simulink model "test_mashinka_mapp_4"  (R2020b)
settings: Solver=ode45  StartTime=0.0  StopTime=20000  RelTol=1e-3  EnableMultiTasking=on
undefined symbols (not defined in the file): CMD_ci_Re_9, CMD_fb, CMD_Firprg_0, CMD_Firprg_1, CMD_gain, CMD_ind_mult, CMD_ind_mult_1, CMD_ind_mult_2, CMD_ind_mult_3, CMD_ind_mult_4, CMD_ind_vol, CMD_ind_vol_1, CMD_ind_vol_2, CMD_ind_vol_3, CMD_ind_vol_4, CMD_nl, CMD_param_0, CMD_pedal, CMD_reset, CMD_shape_0, CMD_step_down, CMD_step_up, ind_mult_0, ind_mult_1, ind_mult_2, ind_mult_3, ind_mult_4, ind_mult_multiplier, num_harm_0, num_pts0, num_str0, num_str1, Res, rom_length
libraries: xbsIndex_r4 x2299
(part 4 of 11)

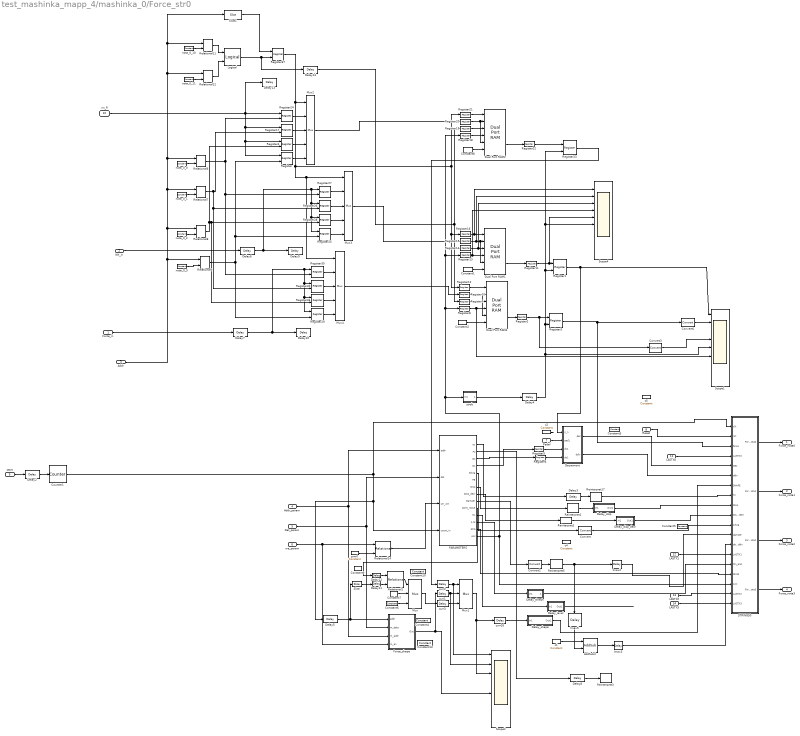
== system test_mashinka_mapp_4/mashinka_0/Force_str0 ==
  Force_in : Inport
  NN_in : Inport  Port=2
  Addr : Inport  Port=3
  Addr_param : Inport  Port=4
  Dat_param : Inport  Port=5
  we_param : Inport  Port=6
  Pedal : Inport  Port=7
  Reset : Inport  Port=8
  start : Inport  Port=9
  nn_fl : Inport  Port=10
  LASTX0 : Inport  Port=11
  LASTX1 : Inport  Port=12
  LASTX2 : Inport  Port=13
  LASTX3 : Inport  Port=14
  AddSub4 : xbsIndex_r4/AddSub  mode=Subtraction  use_carryin=off  use_carryout=off  en=off  latency=4  precision=User Defined  arith_type=Unsigned  n_bits=24  bin_pt=24  quantization=Truncate  overflow=Wrap  use_behavioral_HDL=on  hw_selection=Fabric  pipelined=off  use_rpm=on  dbl_ovrd=off  block_type=addsub
      settings: xl_area=[13 0 0 25 0 0 0]  block_version=VER_STRING_GOES_HERE
  Constant1 : xbsIndex_r4/Constant  const=0  gui_display_data_type=Boolean  arith_type=Boolean  n_bits=48  bin_pt=0  preci_type=Single  exp_width=8  frac_width=24  explicit_period=off  period=1  equ=P=C  opselect=C  inp2=PCIN>>17  opr=+  inp1=P  carry=CIN  dbl_ovrd=off  block_type=constant
      settings: block_version=VER_STRING_GOES_HERE
  Constant10 : xbsIndex_r4/Constant  const=1  gui_display_data_type=Fixed-point  arith_type=Unsigned  n_bits=1  bin_pt=0  preci_type=Single  exp_width=8  frac_width=24  explicit_period=on  period=1  equ=P=C  opselect=C  inp2=PCIN>>17  opr=+  inp1=P  carry=CIN  dbl_ovrd=off  block_type=constant
      settings: block_version=VER_STRING_GOES_HERE
  Constant13 : xbsIndex_r4/Constant  const=0  gui_display_data_type=Fixed-point  arith_type=Unsigned  n_bits=24  bin_pt=0  preci_type=Single  exp_width=8  frac_width=24  explicit_period=on  period=1  equ=P=C  opselect=C  inp2=PCIN>>17  opr=+  inp1=P  carry=CIN  dbl_ovrd=off  block_type=constant
      settings: block_version=VER_STRING_GOES_HERE
  Constant2 : xbsIndex_r4/Constant  const=0  gui_display_data_type=Boolean  arith_type=Boolean  n_bits=48  bin_pt=0  preci_type=Single  exp_width=8  frac_width=24  explicit_period=off  period=1  equ=P=C  opselect=C  inp2=PCIN>>17  opr=+  inp1=P  carry=CIN  dbl_ovrd=off  block_type=constant
      settings: block_version=VER_STRING_GOES_HERE
  Constant3 : xbsIndex_r4/Constant  const=0  gui_display_data_type=Boolean  arith_type=Boolean  n_bits=18  bin_pt=0  preci_type=Single  exp_width=8  frac_width=24  explicit_period=on  period=1  equ=P=C  opselect=C  inp2=PCIN>>17  opr=+  inp1=P  carry=CIN  dbl_ovrd=off  block_type=constant
      settings: block_version=VER_STRING_GOES_HERE
  Constant4 : xbsIndex_r4/Constant  const=100000  gui_display_data_type=Fixed-point  arith_type=Unsigned  n_bits=24  bin_pt=0  preci_type=Single  exp_width=8  frac_width=24  explicit_period=on  period=1  equ=P=C  opselect=C  inp2=PCIN>>17  opr=+  inp1=P  carry=CIN  dbl_ovrd=off  block_type=constant
      settings: block_version=VER_STRING_GOES_HERE
  Constant5 : xbsIndex_r4/Constant  const=1000  gui_display_data_type=Fixed-point  arith_type=Unsigned  n_bits=18  bin_pt=0  preci_type=Single  exp_width=8  frac_width=24  explicit_period=on  period=1  equ=P=C  opselect=C  inp2=PCIN>>17  opr=+  inp1=P  carry=CIN  dbl_ovrd=off  block_type=constant
      settings: block_version=VER_STRING_GOES_HERE
  Constant6 : xbsIndex_r4/Constant  const=1000  gui_display_data_type=Fixed-point  arith_type=Unsigned  n_bits=24  bin_pt=0  preci_type=Single  exp_width=8  frac_width=24  explicit_period=on  period=1  equ=P=C  opselect=C  inp2=PCIN>>17  opr=+  inp1=P  carry=CIN  dbl_ovrd=off  block_type=constant
      settings: block_version=VER_STRING_GOES_HERE
  Constant7 : xbsIndex_r4/Constant  const=0  gui_display_data_type=Fixed-point  arith_type=Unsigned  n_bits=24  bin_pt=0  preci_type=Single  exp_width=8  frac_width=24  explicit_period=on  period=1  equ=P=C  opselect=C  inp2=PCIN>>17  opr=+  inp1=P  carry=CIN  dbl_ovrd=off  block_type=constant
      settings: block_version=VER_STRING_GOES_HERE
  Constant8 : xbsIndex_r4/Constant  const=0  gui_display_data_type=Boolean  arith_type=Boolean  n_bits=48  bin_pt=0  preci_type=Single  exp_width=8  frac_width=24  explicit_period=off  period=1  equ=P=C  opselect=C  inp2=PCIN>>17  opr=+  inp1=P  carry=CIN  dbl_ovrd=off  block_type=constant
      settings: block_version=VER_STRING_GOES_HERE
  Constant9 : xbsIndex_r4/Constant  const=0  gui_display_data_type=Fixed-point  arith_type=Unsigned  n_bits=24  bin_pt=0  preci_type=Single  exp_width=8  frac_width=24  explicit_period=on  period=1  equ=P=C  opselect=C  inp2=PCIN>>17  opr=+  inp1=P  carry=CIN  dbl_ovrd=off  block_type=constant
      settings: block_version=VER_STRING_GOES_HERE
  Convert : xbsIndex_r4/Convert  gui_display_data_type=Fixed-point  arith_type=Unsigned  n_bits=9  bin_pt=0  float_type=Single  exp_bits=8  fraction_bits=24  quantization=Truncate  overflow=Wrap  en=off  latency=0  pipeline=off  dbl_ovrd=off  block_type=convert
  Convert2 : xbsIndex_r4/Convert  gui_display_data_type=Fixed-point  arith_type=Unsigned  n_bits=24  bin_pt=0  float_type=Single  exp_bits=8  fraction_bits=24  quantization=Truncate  overflow=Wrap  en=off  latency=0  pipeline=off  dbl_ovrd=off  block_type=convert
      settings: block_version=VER_STRING_GOES_HERE
  Convert3 : xbsIndex_r4/Convert  gui_display_data_type=Floating-point  arith_type=Floating-point  n_bits=16  bin_pt=14  float_type=Single  exp_bits=8  fraction_bits=24  quantization=Truncate  overflow=Wrap  en=off  latency=0  pipeline=off  dbl_ovrd=off  block_type=convert
  Convert6 : xbsIndex_r4/Convert  gui_display_data_type=Floating-point  arith_type=Floating-point  n_bits=16  bin_pt=14  float_type=Single  exp_bits=8  fraction_bits=24  quantization=Truncate  overflow=Wrap  en=off  latency=0  pipeline=off  dbl_ovrd=off  block_type=convert
  Counter1 : xbsIndex_r4/Counter  cnt_type=Count Limited  cnt_to=num_str0*(num_point_256) - 1  operation=Up  start_count=0  cnt_by_val=1  arith_type=Unsigned  n_bits=ceil(log2(num_str0*num_point_256))  bin_pt=0  load_pin=off  rst=off  en=on  explicit_period=on  period=1  use_behavioral_HDL=off  implementation=Fabric  use_rpm=off  dbl_ovrd=off  block_type=counter
      settings: block_version=8.2.02
  Decrement : Subsystem
  Delay10 : xbsIndex_r4/Delay  rst=off  infoeditControl=Selection of Reset will increase slice count due to use of real FFs and instead of SRLs  en=off  latency=5  reg_retiming=on  dbl_ovrd=off  block_type=delay
      settings: xl_area=[2 4 0 4 0 0 0]  block_version=8.2-EVAL
  Delay{2,6,11..12,14} (5 alike) : xbsIndex_r4/Delay  rst=off  infoeditControl=Selection of Reset will increase slice count due to use of real FFs and instead of SRLs  en=off  latency=1  reg_retiming=on  dbl_ovrd=off  block_type=delay
      settings: xl_area=[2 4 0 4 0 0 0]  block_version=8.2-EVAL
  Delay13 : xbsIndex_r4/Delay  rst=off  infoeditControl=Selection of Reset will increase slice count due to use of real FFs and instead of SRLs  en=off  latency=6  reg_retiming=on  dbl_ovrd=off  block_type=delay
      settings: xl_area=[2 4 0 4 0 0 0]  block_version=8.2-EVAL
  Delay3 : xbsIndex_r4/Delay  rst=off  infoeditControl=Selection of Reset will increase slice count due to use of real FFs and instead of SRLs  en=off  latency=29  reg_retiming=on  dbl_ovrd=off  block_type=delay
      settings: xl_area=[2 4 0 4 0 0 0]  block_version=8.2-EVAL
  Delay4 : xbsIndex_r4/Delay  rst=off  infoeditControl=Selection of Reset will increase slice count due to use of real FFs and instead of SRLs  en=off  latency=3  reg_retiming=on  dbl_ovrd=off  block_type=delay
      settings: xl_area=[2 4 0 4 0 0 0]  block_version=8.2-EVAL
  Delay5 : xbsIndex_r4/Delay  rst=off  infoeditControl=Selection of Reset will increase slice count due to use of real FFs and instead of SRLs  en=off  latency=23  reg_retiming=on  dbl_ovrd=off  block_type=delay
      settings: xl_area=[2 4 0 4 0 0 0]  block_version=8.2-EVAL
  Delay7 : xbsIndex_r4/Delay  rst=off  infoeditControl=Selection of Reset will increase slice count due to use of real FFs and instead of SRLs  en=off  latency=2  reg_retiming=on  dbl_ovrd=off  block_type=delay
      settings: xl_area=[2 4 0 4 0 0 0]  block_version=8.2-EVAL
  Delay8 : xbsIndex_r4/Delay  rst=off  infoeditControl=Selection of Reset will increase slice count due to use of real FFs and instead of SRLs  en=off  latency=28  reg_retiming=on  dbl_ovrd=off  block_type=delay
      settings: xl_area=[2 4 0 4 0 0 0]  block_version=8.2-EVAL
  Delay9 : xbsIndex_r4/Delay  rst=off  infoeditControl=Selection of Reset will increase slice count due to use of real FFs and instead of SRLs  en=off  latency=5  reg_retiming=on  dbl_ovrd=off  block_type=delay
      settings: xl_area=[2 4 0 4 0 0 0]  block_version=8.2-EVAL
  Delay_disp : Subsystem
  Delay_disp_decr : Subsystem
  Delay_level : Subsystem
  Delay_shape : Subsystem
  Delay_thresh : Subsystem
  Dual Port RAM1 : xbsIndex_r4/Dual Port RAM  depth=2^ceil(log2(num_str1))  initVector=zeros  distributed_mem=Block RAM  init_a=0  init_b=0  rst_a=off  rst_b=off  en_a=off  en_b=off  latency=1  write_mode_A=Read Before Write  write_mode_B=Read Before Write  optimize=Area  dbl_ovrd=off  simulation_type=fast_sim  block_type=dpram
      settings: block_version=10.1.1
  Dual Port RAM2 : xbsIndex_r4/Dual Port RAM  depth=2^ceil(log2(num_str1))  initVector=zeros  distributed_mem=Block RAM  init_a=0  init_b=0  rst_a=off  rst_b=off  en_a=off  en_b=off  latency=1  write_mode_A=Read Before Write  write_mode_B=Read Before Write  optimize=Area  dbl_ovrd=off  simulation_type=fast_sim  block_type=dpram
      settings: block_version=10.1.1
  Dual Port RAM4 : xbsIndex_r4/Dual Port RAM  depth=2^ceil(log2(num_str1))  initVector=zeros  distributed_mem=Block RAM  init_a=0  init_b=0  rst_a=off  rst_b=off  en_a=off  en_b=off  latency=1  write_mode_A=Read Before Write  write_mode_B=Read Before Write  optimize=Area  dbl_ovrd=off  simulation_type=fast_sim  block_type=dpram
      settings: block_version=10.1.1
  Force_shape : Subsystem
  Imax2 : xbsIndex_r4/Delay  rst=off  infoeditControl=Selection of Reset will increase slice count due to use of real FFs and instead of SRLs  en=off  latency=1  reg_retiming=on  dbl_ovrd=off  block_type=delay
      settings: xl_area=[12 24 0 0 0 0 0]  block_version=VER_STRING_GOES_HERE
  Imax3 : xbsIndex_r4/Delay  rst=off  infoeditControl=Selection of Reset will increase slice count due to use of real FFs and instead of SRLs  en=off  latency=1  reg_retiming=on  dbl_ovrd=off  block_type=delay
      settings: xl_area=[12 24 0 0 0 0 0]  block_version=VER_STRING_GOES_HERE
  Imax5 : xbsIndex_r4/Delay  rst=off  infoeditControl=Selection of Reset will increase slice count due to use of real FFs and instead of SRLs  en=off  latency=6  reg_retiming=on  dbl_ovrd=off  block_type=delay
      settings: infoedit=Hardware notes: A delay line is a chain, each link of which is an SRL16 followed by a flip-flop. If register retiming is enabled, the delay line is a chain of flip-flops.  xl_area=[12 24 0 24 0 0 0]  block_version=VER_STRING_GOES_HERE
  Logical : xbsIndex_r4/Logical  logical_function=AND  inputs=2  en=off  latency=0  precision=Full  arith_type=Unsigned  n_bits=16  bin_pt=0  align_bp=on  dbl_ovrd=off  block_type=logical
  Mux : xbsIndex_r4/Mux  inputs=2  en=off  latency=1  precision=Full  arith_type=Unsigned  n_bits=16  bin_pt=14  quantization=Truncate  overflow=Wrap  dbl_ovrd=off  block_type=mux
  Mux1 : xbsIndex_r4/Mux  inputs=2  en=off  latency=0  precision=Full  arith_type=Unsigned  n_bits=16  bin_pt=14  quantization=Truncate  overflow=Wrap  dbl_ovrd=off  block_type=mux
  Mux2 : xbsIndex_r4/Mux  inputs=4  en=off  latency=0  precision=Full  arith_type=Unsigned  n_bits=16  bin_pt=14  quantization=Truncate  overflow=Wrap  dbl_ovrd=off  block_type=mux
  Mux3 : xbsIndex_r4/Mux  inputs=4  en=off  latency=0  precision=Full  arith_type=Unsigned  n_bits=16  bin_pt=14  quantization=Truncate  overflow=Wrap  dbl_ovrd=off  block_type=mux
  Mux4 : xbsIndex_r4/Mux  inputs=4  en=off  latency=0  precision=Full  arith_type=Unsigned  n_bits=16  bin_pt=14  quantization=Truncate  overflow=Wrap  dbl_ovrd=off  block_type=mux
  PARAMETERS : Subsystem
  Register{,1,3..4,17,23..30,35..37} (16 alike) : xbsIndex_r4/Register  init=0  rst=off  en=on  dbl_ovrd=off  block_type=register
      Register1 settings: xl_area=[18 36 0 0 0 0 0]  block_version=VER_STRING_GOES_HERE
      Register23 settings: xl_area=[18 36 0 0 0 0 0]  block_version=VER_STRING_GOES_HERE
      Register3 settings: xl_area=[18 36 0 0 0 0 0]  block_version=VER_STRING_GOES_HERE
  Register{2,5..6,8..16,18..22} (17 alike) : xbsIndex_r4/Register  init=0  rst=off  en=off  dbl_ovrd=off  block_type=register
  Reinterpret{1..3,17} (4 alike) : xbsIndex_r4/Reinterpret  force_arith_type=off  arith_type="Signed  (2's comp)"  force_bin_pt=on  bin_pt=24  block_type=cast
      settings: block_version=VER_STRING_GOES_HERE
  Reinterpret5 : xbsIndex_r4/Reinterpret  force_arith_type=on  arith_type=Unsigned  force_bin_pt=on  bin_pt=24  block_type=cast
      settings: block_version=VER_STRING_GOES_HERE
  Relational{1,6..9,14} (6 alike) : xbsIndex_r4/Relational  mode=a=b  op_type=Bool  en=off  latency=0  dbl_ovrd=off  block_type=relational
      Relational6 settings: block_version=9.2.01
      Relational7 settings: block_version=9.2.01
      Relational8 settings: block_version=9.2.01
      Relational9 settings: block_version=9.2.01
  Relational11 : xbsIndex_r4/Relational  mode=a<=b  op_type=Bool  en=off  latency=0  dbl_ovrd=off  block_type=relational
      settings: block_version=9.2.01
  Relational12 : xbsIndex_r4/Relational  mode=a>b  op_type=Bool  en=off  latency=0  dbl_ovrd=off  block_type=relational
      settings: block_version=9.2.01
  STRINGS0 : Subsystem
  Scope1 : Scope  NumInputPorts=9
  Scope2 : Scope  NumInputPorts=8
  Scope4 : Scope  NumInputPorts=10
  Slice : xbsIndex_r4/Slice  nbits=8  boolean_output=off  mode=Lower Bit Location + Width  bit1=0  base1=MSB of Input  bit0=0  base0=LSB of Input  dbl_ovrd=off  block_type=slice
  Slice1 : xbsIndex_r4/Slice  nbits=2  boolean_output=off  mode=Lower Bit Location + Width  bit1=0  base1=MSB of Input  bit0=0  base0=LSB of Input  dbl_ovrd=off  block_type=slice
  c1 : xbsIndex_r4/Constant  const=1  gui_display_data_type=Fixed-point  arith_type=Unsigned  n_bits=24  bin_pt=23  preci_type=Single  exp_width=8  frac_width=24  explicit_period=off  period=1  equ=P=C  opselect=C  inp2=PCIN>>17  opr=+  inp1=P  carry=CIN  dbl_ovrd=off  block_type=constant
      settings: block_version=VER_STRING_GOES_HERE
  c2 : xbsIndex_r4/Constant  const=0  gui_display_data_type=Fixed-point  arith_type=Unsigned  n_bits=7  bin_pt=0  preci_type=Single  exp_width=8  frac_width=24  explicit_period=off  period=1  equ=P=C  opselect=C  inp2=PCIN>>17  opr=+  inp1=P  carry=CIN  dbl_ovrd=off  block_type=constant
      settings: block_version=VER_STRING_GOES_HERE
  c4 : xbsIndex_r4/Constant  const=200  gui_display_data_type=Fixed-point  arith_type=Unsigned  n_bits=8  bin_pt=0  preci_type=Single  exp_width=8  frac_width=24  explicit_period=on  period=1  equ=P=C  opselect=C  inp2=PCIN>>17  opr=+  inp1=P  carry=CIN  dbl_ovrd=off  block_type=constant
      settings: block_version=VER_STRING_GOES_HERE
  c5 : xbsIndex_r4/Constant  const=0  gui_display_data_type=Fixed-point  arith_type=Unsigned  n_bits=7  bin_pt=0  preci_type=Single  exp_width=8  frac_width=24  explicit_period=off  period=1  equ=P=C  opselect=C  inp2=PCIN>>17  opr=+  inp1=P  carry=CIN  dbl_ovrd=off  block_type=constant
      settings: block_version=VER_STRING_GOES_HERE
  curr{1..3,16} (4 alike) : xbsIndex_r4/Delay  rst=off  infoeditControl=Selection of Reset will increase slice count due to use of real FFs and instead of SRLs  en=off  latency=1  reg_retiming=on  dbl_ovrd=off  block_type=delay
      settings: xl_area=[17 33 0 33 0 0 0]  block_version=VER_STRING_GOES_HERE
  nota_0_0 : xbsIndex_r4/Constant  const=nota_0_0  gui_display_data_type=Fixed-point  arith_type=Unsigned  n_bits=7  bin_pt=0  preci_type=Single  exp_width=8  frac_width=24  explicit_period=on  period=1  equ=P=C  opselect=C  inp2=PCIN>>17  opr=+  inp1=P  carry=CIN  dbl_ovrd=off  block_type=constant
      settings: block_version=VER_STRING_GOES_HERE
  nota_0_1 : xbsIndex_r4/Constant  const=nota_0_1  gui_display_data_type=Fixed-point  arith_type=Unsigned  n_bits=7  bin_pt=0  preci_type=Single  exp_width=8  frac_width=24  explicit_period=on  period=1  equ=P=C  opselect=C  inp2=PCIN>>17  opr=+  inp1=P  carry=CIN  dbl_ovrd=off  block_type=constant
      settings: block_version=VER_STRING_GOES_HERE
  nota_0_10 : xbsIndex_r4/Constant  const=95  gui_display_data_type=Fixed-point  arith_type=Unsigned  n_bits=7  bin_pt=0  preci_type=Single  exp_width=8  frac_width=24  explicit_period=on  period=1  equ=P=C  opselect=C  inp2=PCIN>>17  opr=+  inp1=P  carry=CIN  dbl_ovrd=off  block_type=constant
      settings: block_version=VER_STRING_GOES_HERE
  nota_0_11 : xbsIndex_r4/Constant  const=91  gui_display_data_type=Fixed-point  arith_type=Unsigned  n_bits=7  bin_pt=0  preci_type=Single  exp_width=8  frac_width=24  explicit_period=on  period=1  equ=P=C  opselect=C  inp2=PCIN>>17  opr=+  inp1=P  carry=CIN  dbl_ovrd=off  block_type=constant
      settings: block_version=VER_STRING_GOES_HERE
  nota_0_2 : xbsIndex_r4/Constant  const=nota_0_2  gui_display_data_type=Fixed-point  arith_type=Unsigned  n_bits=7  bin_pt=0  preci_type=Single  exp_width=8  frac_width=24  explicit_period=on  period=1  equ=P=C  opselect=C  inp2=PCIN>>17  opr=+  inp1=P  carry=CIN  dbl_ovrd=off  block_type=constant
      settings: block_version=VER_STRING_GOES_HERE
  nota_0_3 : xbsIndex_r4/Constant  const=nota_0_3  gui_display_data_type=Fixed-point  arith_type=Unsigned  n_bits=7  bin_pt=0  preci_type=Single  exp_width=8  frac_width=24  explicit_period=on  period=1  equ=P=C  opselect=C  inp2=PCIN>>17  opr=+  inp1=P  carry=CIN  dbl_ovrd=off  block_type=constant
      settings: block_version=VER_STRING_GOES_HERE
  prm0 : xbsIndex_r4/Constant  const=prm0  gui_display_data_type=Fixed-point  arith_type=Unsigned  n_bits=8  bin_pt=0  preci_type=Single  exp_width=8  frac_width=24  explicit_period=on  period=1  equ=P=C  opselect=C  inp2=PCIN>>17  opr=+  inp1=P  carry=CIN  dbl_ovrd=off  block_type=constant
      settings: block_version=VER_STRING_GOES_HERE
  strob : Subsystem
  Force_nota0 : Outport  VectorParamsAs1DForOutWhenUnconnected=off
  Force_nota1 : Outport  Port=2  VectorParamsAs1DForOutWhenUnconnected=off
  Force_nota2 : Outport  Port=3  VectorParamsAs1DForOutWhenUnconnected=off
  Force_nota3 : Outport  Port=4  VectorParamsAs1DForOutWhenUnconnected=off
  wires:
  Mux/1 -> curr3/1
  strob/1(Out1) -> Delay4/1
  Register23/1 -> curr2/1
  Register22/1 -> Register23/1
  Dual Port RAM2/2 -> Register22/1
  Mux2/1 -> Register20/1
  Register21/1 -> Dual Port RAM2/1
  Register20/1 -> Dual Port RAM2/5, Dual Port RAM2/2
  Register19/1 -> Dual Port RAM2/3
  Constant8/1 -> Dual Port RAM2/6
  nn_fl/1 -> Register/1, Register4/1, Register17/1, Delay13/1, Register24/1
  curr3/1 -> Mux1/3
  curr1/1 -> Mux1/2, Scope2/2
  curr2/1 -> Mux1/1, Scope2/1
  curr16/1 -> Delay_shape/1(In1)
  Slice/1 -> Delay11/1
  Delay12/1 -> Relational1/1
  Constant7/1 -> Mux/2
  Constant6/1 -> Mux/3
  Relational1/1 -> Mux/1
  PARAMETERS/10(point_noise) -> Delay12/1
  Delay11/1 -> Relational1/2
  PARAMETERS/11(NL) -> Delay_level/1(In1)
  LASTX1/1 -> STRINGS0/14(LASTX1)
  Mux4/1 -> Register10/1
  NN_in/1 -> Delay6/1
  Convert/1 -> STRINGS0/11(sdvig)
  PARAMETERS/2(Fo) -> Delay8/1
  Delay8/1 -> Reinterpret3/1
  PARAMETERS/14(Acc) -> STRINGS0/17(Acc), Register13/1, Register18/1, Register8/1, strob/1(In1)
  Constant1/1 -> Dual Port RAM1/6
  Constant2/1 -> Dual Port RAM4/6
  Dual Port RAM4/2 -> Register2/1
  Delay14/1 -> Register9/1, Register14/1, Register19/1
  c2/1 -> ?
  PARAMETERS/4(Dc) -> Register5/1
  PARAMETERS/3(Do) -> Register6/1
  Dual Port RAM1/2 -> Register11/1
  Decrement/1(dec) -> STRINGS0/5(Dec)
  PARAMETERS/7(Disp) -> Reinterpret1/1
  PARAMETERS/8(Disp_decr) -> Reinterpret2/1
  Mux1/1 -> Scope2/3, curr16/1
  Reinterpret17/1 -> STRINGS0/8(Tn)
  Reinterpret1/1 -> Delay_disp/1(In1)
  Reinterpret2/1 -> Delay_disp_decr/1(In1)
  PARAMETERS/1(Tn) -> Delay3/1
  Delay3/1 -> Reinterpret17/1
  Decrement/2(ddiv) -> STRINGS0/6(ddiv)
  PARAMETERS/5(Sdvig) -> Convert/1
  Addr_param/1 -> Force_shape/3(m_addr), PARAMETERS/1(addr)
  Dat_param/1 -> Force_shape/2(m_data), PARAMETERS/2(dat)
  we_param/1 -> Relational14/1, Force_shape/4(m_en)
  Pedal/1 -> Decrement/2(ped1)
  Reset/1 -> STRINGS0/2(rst)
  LASTX0/1 -> STRINGS0/4(LASTX0)
  Force_in/1 -> Delay7/1
  Delay5/1 -> Force_shape/1(addr), Slice/1
  Register11/1 -> Scope4/5, Register1/1
  Register2/1 -> Convert3/1, Register3/1
  Register5/1 -> Decrement/3(dc1)
  Register6/1 -> Decrement/4(do1)
  Register1/1 -> Decrement/1(n_n), Scope1/1
  Register8/1 -> Scope1/6, Dual Port RAM4/4
  Register10/1 -> Dual Port RAM4/2, Dual Port RAM4/5
  Register12/1 -> Dual Port RAM4/1
  Register13/1 -> Dual Port RAM1/4, Scope4/4
  Register14/1 -> Scope4/3, Dual Port RAM1/3
  Register15/1 -> Scope4/2, Dual Port RAM1/2, Dual Port RAM1/5
  Register16/1 -> Scope4/1, Dual Port RAM1/1
  Convert2/1 -> Reinterpret5/1
  AddSub4/1 -> Imax3/1
  c1/1 -> AddSub4/1
  Reinterpret5/1 -> Imax5/1, Imax2/1
  Imax5/1 -> AddSub4/2
  Imax2/1 -> STRINGS0/12(damper)
  Imax3/1 -> STRINGS0/13(damper_ddiv)
  PARAMETERS/9(Damper) -> Convert2/1
  prm0/1 -> Relational14/2
  Relational14/1 -> PARAMETERS/3(str_we)
  Delay2/1 -> Counter1/1
  start/1 -> Delay2/1
  PARAMETERS/12(1-Nl) -> Delay_thresh/1(In1)
  Delay_thresh/1(ttn_end) -> STRINGS0/15(ttn_end)
  Delay_level/1(Out1) -> ?
  Delay_disp/1(Out1) -> STRINGS0/9(Disp)
  Delay_disp_decr/1(Out1) -> STRINGS0/10(Disp_decr)
  Delay_shape/1(Out1) -> STRINGS0/7(SHAPE)
  Mux3/1 -> Register15/1
  Register3/1 -> STRINGS0/3(force), Convert6/1
  Force_shape/1(Out) -> curr1/1, Scope2/5
  Register37/1 -> Mux4/1, Mux3/1, Register12/1, Register16/1, Register21/1, Mux2/1
  Register9/1 -> Dual Port RAM4/3
  PARAMETERS/13(Strb) -> STRINGS0/16(Strob)
  Register18/1 -> Dual Port RAM2/4
  Delay4/1 -> Scope1/5, Register1/2, Scope4/6, Register23/2, Register3/2
  Counter1/1 -> Delay5/1, PARAMETERS/4(count_in), STRINGS0/1(clk)
  STRINGS0/2(Force_nota1) -> Force_nota1/1
  STRINGS0/1(Force_nota0) -> Force_nota0/1
  STRINGS0/3(Force_nota2) -> Force_nota2/1
  STRINGS0/4(Force_nota3) -> Force_nota3/1
  LASTX2/1 -> STRINGS0/18(LASTX2)
  LASTX3/1 -> STRINGS0/19(LASTX3)
  Convert6/1 -> Scope1/2
  Convert3/1 -> Scope1/4
  nota_0_2/1 -> Relational8/2
  nota_0_3/1 -> Relational9/2
  nota_0_1/1 -> Relational7/2
  nota_0_0/1 -> Relational6/2
  Delay7/1 -> Register30/1, Register36/1, Register29/1, Register35/1, Delay10/1
  Relational6/1 -> Register35/2, Register27/2, Register24/2
  Relational7/1 -> Register30/2, Register26/2, Register17/2
  Relational8/1 -> Register36/2, Register28/2, Register4/2
  Relational9/1 -> Register29/2, Register25/2, Register/2
  Register24/1 -> Mux2/2
  Register17/1 -> Mux2/3
  Register4/1 -> Mux2/4
  Register/1 -> Mux2/5
  Register27/1 -> Mux3/2
  Register26/1 -> Mux3/3
  Register28/1 -> Mux3/4
  Register25/1 -> Mux3/5
  Register35/1 -> Mux4/2
  Register30/1 -> Mux4/3
  Register36/1 -> Mux4/4
  Register29/1 -> Mux4/5
  nota_0_10/1 -> Relational11/2
  nota_0_11/1 -> Relational12/2
  Addr/1 -> Slice1/1, Relational11/1, Relational12/1, Relational6/1, Relational7/1, Relational8/1, Relational9/1
  Relational11/1 -> Logical/1
  Relational12/1 -> Logical/2
  Logical/1 -> Delay14/1, Register37/2
  Slice1/1 -> Register37/1
  Delay6/1 -> Register26/1, Register28/1, Register25/1, Register27/1, Delay9/1

== system test_mashinka_mapp_4/Mid_Graph1/Exp/exp-mashinka ==
  Force_vol : Inport
  m_data : Inport  Port=2
  m_addr : Inport  Port=3
  m_en : Inport  Port=4
  Addr_ind_vol : Inport  Port=5
  Addr_sync : Inport  Port=6
  AddSub : xbsIndex_r4/AddSub  mode=Addition  use_carryin=off  use_carryout=off  en=off  latency=8  precision=Full  arith_type=Unsigned  n_bits=16  bin_pt=14  quantization=Truncate  overflow=Wrap  use_behavioral_HDL=off  hw_selection=Fabric  pipelined=off  dbl_ovrd=off  block_type=addsub
  AddSub1 : xbsIndex_r4/AddSub  mode=Addition  use_carryin=off  use_carryout=off  en=off  latency=8  precision=Full  arith_type=Unsigned  n_bits=16  bin_pt=14  quantization=Truncate  overflow=Wrap  use_behavioral_HDL=off  hw_selection=Fabric  pipelined=off  dbl_ovrd=off  block_type=addsub
  AddSub2 : xbsIndex_r4/AddSub  mode=Addition  use_carryin=off  use_carryout=off  en=off  latency=8  precision=Full  arith_type=Unsigned  n_bits=16  bin_pt=14  quantization=Truncate  overflow=Wrap  use_behavioral_HDL=off  hw_selection=Fabric  pipelined=off  dbl_ovrd=off  block_type=addsub
  Constant : xbsIndex_r4/Constant  const=0  gui_display_data_type=Fixed-point  arith_type=Unsigned  n_bits=30  bin_pt=0  preci_type=Single  exp_width=8  frac_width=24  explicit_period=on  period=1  equ=P=C  opselect=C  inp2=PCIN>>17  opr=+  inp1=P  carry=CIN  dbl_ovrd=off  block_type=constant
  Convert5 : xbsIndex_r4/Convert  gui_display_data_type=Floating-point  arith_type=Floating-point  n_bits=16  bin_pt=14  float_type=Single  exp_bits=8  fraction_bits=24  quantization=Truncate  overflow=Wrap  en=off  latency=0  pipeline=off  dbl_ovrd=off  block_type=convert
  Convert6 : xbsIndex_r4/Convert  gui_display_data_type=Floating-point  arith_type=Floating-point  n_bits=16  bin_pt=14  float_type=Single  exp_bits=8  fraction_bits=24  quantization=Truncate  overflow=Wrap  en=off  latency=0  pipeline=off  dbl_ovrd=off  block_type=convert
  Convert7 : xbsIndex_r4/Convert  gui_display_data_type=Floating-point  arith_type=Floating-point  n_bits=16  bin_pt=14  float_type=Single  exp_bits=8  fraction_bits=24  quantization=Truncate  overflow=Wrap  en=off  latency=0  pipeline=off  dbl_ovrd=off  block_type=convert
  Delay : xbsIndex_r4/Delay  rst=off  infoeditControl=Selection of Reset will increase slice count due to use of real FFs and instead of SRLs  en=off  latency=50  reg_retiming=off  dbl_ovrd=off  block_type=delay
  Delay1 : xbsIndex_r4/Delay  rst=off  infoeditControl=Selection of Reset will increase slice count due to use of real FFs and instead of SRLs  en=off  latency=1  reg_retiming=off  dbl_ovrd=off  block_type=delay
  Delay11 : xbsIndex_r4/Delay  rst=off  infoeditControl=Selection of Reset will increase slice count due to use of real FFs and instead of SRLs  en=off  latency=1  reg_retiming=off  dbl_ovrd=off  block_type=delay
  Delay2 : xbsIndex_r4/Delay  rst=off  infoeditControl=Selection of Reset will increase slice count due to use of real FFs and instead of SRLs  en=off  latency=1  reg_retiming=off  dbl_ovrd=off  block_type=delay
  Relational : xbsIndex_r4/Relational  mode=a!=b  op_type=Bool  en=off  latency=1  dbl_ovrd=off  block_type=relational
  Scope3 : Scope  NumInputPorts=10
  gauss0 : Subsystem
  gauss1 : Subsystem
  gauss2 : Subsystem
  gauss3 : Subsystem
  z12 : xbsIndex_r4/Delay  rst=off  infoeditControl=Selection of Reset will increase slice count due to use of real FFs and instead of SRLs  en=off  latency=1  reg_retiming=on  dbl_ovrd=off  block_type=delay
      settings: block_version=8.2-EVAL
  z9 : xbsIndex_r4/Delay  rst=off  infoeditControl=Selection of Reset will increase slice count due to use of real FFs and instead of SRLs  en=off  latency=1  reg_retiming=on  dbl_ovrd=off  block_type=delay
      settings: block_version=8.2-EVAL
  Out : Outport  VectorParamsAs1DForOutWhenUnconnected=off
  wires:
  AddSub2/1 -> Delay1/1
  Delay1/1 -> AddSub1/2
  gauss3/1(Out1) -> AddSub2/2
  gauss2/1(Out1) -> AddSub2/1
  gauss1/1(Out1) -> AddSub/2
  Convert7/1 -> Scope3/7
  Convert5/1 -> Scope3/5
  AddSub1/1 -> Delay2/1, Convert7/1
  AddSub/1 -> Delay11/1
  Delay11/1 -> Convert5/1, AddSub1/1
  gauss0/1(Out1) -> Convert6/1, AddSub/1
  z9/1 -> gauss0/7(Addr_ind_vol), gauss2/7(Addr_ind_vol), gauss3/7(Addr_ind_vol), gauss1/7(Addr_ind_vol)
  m_en/1 -> gauss0/6(m_en), gauss2/6(m_en), gauss3/6(m_en), gauss1/6(m_en)
  m_addr/1 -> gauss0/5(m_addr), gauss2/5(m_addr), gauss3/5(m_addr), gauss1/5(m_addr)
  m_data/1 -> gauss0/4(m_data), gauss2/4(m_data), gauss3/4(m_data), gauss1/4(m_data)
  Force_vol/1 -> gauss2/3(Force_vol), gauss3/3(Force_vol), gauss1/3(Force_vol), gauss0/3(Force_vol)
  Delay/1 -> gauss2/1(sync), gauss3/1(sync), gauss1/1(sync), gauss0/1(sync)
  z12/1 -> Relational/1, gauss0/2(addr), gauss2/2(addr), gauss3/2(addr), gauss1/2(addr)
  Delay2/1 -> Out/1
  Convert6/1 -> Scope3/1
  Relational/1 -> Delay/1
  Constant/1 -> Relational/2
  Addr_ind_vol/1 -> z9/1
  Addr_sync/1 -> z12/1

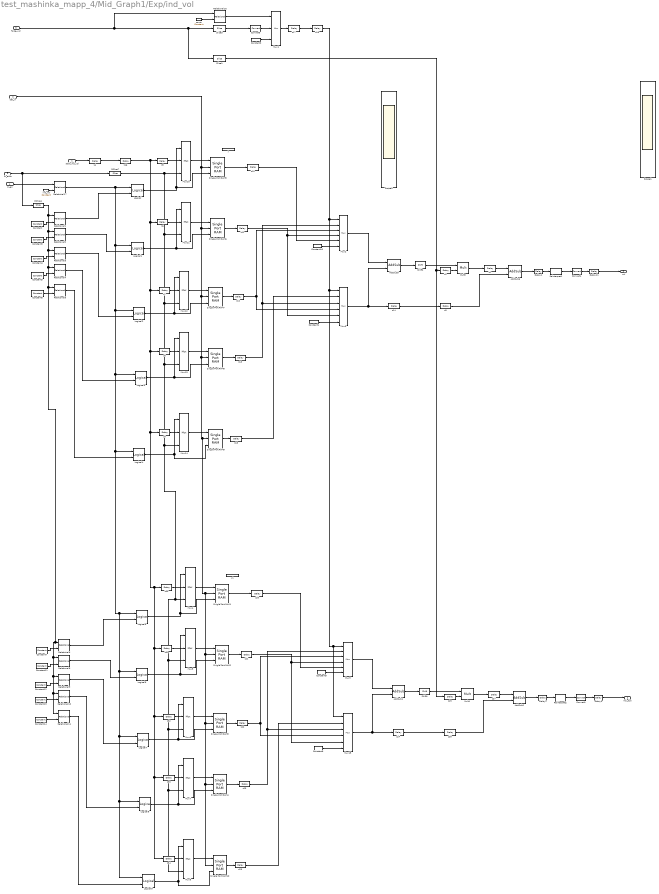
== system test_mashinka_mapp_4/Mid_Graph1/Exp/ind_vol ==
  addr_ind_vol : Inport
  dat_in : Inport  Port=2
  m_addr : Inport  Port=3
  m_en : Inport  Port=4
  force_vol : Inport  Port=5
  AddSub1 : xbsIndex_r4/AddSub  mode=Subtraction  use_carryin=off  use_carryout=off  en=off  latency=2  precision=Full  arith_type="Signed  (2's comp)"  n_bits=24  bin_pt=0  quantization=Truncate  overflow=Wrap  use_behavioral_HDL=off  hw_selection=Fabric  pipelined=off  dbl_ovrd=off  block_type=addsub
  AddSub2 : xbsIndex_r4/AddSub  mode=Addition  use_carryin=off  use_carryout=off  en=off  latency=2  precision=Full  arith_type=Unsigned  n_bits=24  bin_pt=0  quantization=Truncate  overflow=Wrap  use_behavioral_HDL=off  hw_selection=Fabric  pipelined=off  dbl_ovrd=off  block_type=addsub
  AddSub5 : xbsIndex_r4/AddSub  mode=Subtraction  use_carryin=off  use_carryout=off  en=off  latency=2  precision=Full  arith_type="Signed  (2's comp)"  n_bits=24  bin_pt=0  quantization=Truncate  overflow=Wrap  use_behavioral_HDL=off  hw_selection=Fabric  pipelined=off  dbl_ovrd=off  block_type=addsub
  AddSub6 : xbsIndex_r4/AddSub  mode=Addition  use_carryin=off  use_carryout=off  en=off  latency=2  precision=Full  arith_type=Unsigned  n_bits=24  bin_pt=0  quantization=Truncate  overflow=Wrap  use_behavioral_HDL=off  hw_selection=Fabric  pipelined=off  dbl_ovrd=off  block_type=addsub
  Constant : xbsIndex_r4/Constant  const=4  gui_display_data_type=Fixed-point  arith_type=Unsigned  n_bits=3  bin_pt=0  preci_type=Single  exp_width=8  frac_width=24  explicit_period=off  period=1  equ=P=C  opselect=C  inp2=PCIN>>17  opr=+  inp1=P  carry=CIN  dbl_ovrd=off  block_type=constant
  Constant{1,8..10} (4 alike) : xbsIndex_r4/Constant  const=0  gui_display_data_type=Fixed-point  arith_type=Unsigned  n_bits=24  bin_pt=0  preci_type=Single  exp_width=8  frac_width=24  explicit_period=on  period=1  equ=P=C  opselect=C  inp2=PCIN>>17  opr=+  inp1=P  carry=CIN  dbl_ovrd=off  block_type=constant
      settings: block_version=VER_STRING_GOES_HERE
  Constant11 : xbsIndex_r4/Constant  const=8  gui_display_data_type=Fixed-point  arith_type=Unsigned  n_bits=4  bin_pt=0  preci_type=Single  exp_width=8  frac_width=24  explicit_period=off  period=1  equ=P=C  opselect=C  inp2=PCIN>>17  opr=+  inp1=P  carry=CIN  dbl_ovrd=off  block_type=constant
  Constant12 : xbsIndex_r4/Constant  const=7  gui_display_data_type=Fixed-point  arith_type=Unsigned  n_bits=4  bin_pt=0  preci_type=Single  exp_width=8  frac_width=24  explicit_period=off  period=1  equ=P=C  opselect=C  inp2=PCIN>>17  opr=+  inp1=P  carry=CIN  dbl_ovrd=off  block_type=constant
  Constant13 : xbsIndex_r4/Constant  const=6  gui_display_data_type=Fixed-point  arith_type=Unsigned  n_bits=4  bin_pt=0  preci_type=Single  exp_width=8  frac_width=24  explicit_period=off  period=1  equ=P=C  opselect=C  inp2=PCIN>>17  opr=+  inp1=P  carry=CIN  dbl_ovrd=off  block_type=constant
  Constant14 : xbsIndex_r4/Constant  const=5  gui_display_data_type=Fixed-point  arith_type=Unsigned  n_bits=4  bin_pt=0  preci_type=Single  exp_width=8  frac_width=24  explicit_period=off  period=1  equ=P=C  opselect=C  inp2=PCIN>>17  opr=+  inp1=P  carry=CIN  dbl_ovrd=off  block_type=constant
  Constant2 : xbsIndex_r4/Constant  const=4  gui_display_data_type=Fixed-point  arith_type=Unsigned  n_bits=3  bin_pt=0  preci_type=Single  exp_width=8  frac_width=24  explicit_period=on  period=1  equ=P=C  opselect=C  inp2=PCIN>>17  opr=+  inp1=P  carry=CIN  dbl_ovrd=off  block_type=constant
      settings: block_version=VER_STRING_GOES_HERE
  Constant3 : xbsIndex_r4/Constant  const=3  gui_display_data_type=Fixed-point  arith_type=Unsigned  n_bits=3  bin_pt=0  preci_type=Single  exp_width=8  frac_width=24  explicit_period=off  period=1  equ=P=C  opselect=C  inp2=PCIN>>17  opr=+  inp1=P  carry=CIN  dbl_ovrd=off  block_type=constant
  Constant4 : xbsIndex_r4/Constant  const=2  gui_display_data_type=Fixed-point  arith_type=Unsigned  n_bits=3  bin_pt=0  preci_type=Single  exp_width=8  frac_width=24  explicit_period=off  period=1  equ=P=C  opselect=C  inp2=PCIN>>17  opr=+  inp1=P  carry=CIN  dbl_ovrd=off  block_type=constant
  Constant5 : xbsIndex_r4/Constant  const=1  gui_display_data_type=Fixed-point  arith_type=Unsigned  n_bits=3  bin_pt=0  preci_type=Single  exp_width=8  frac_width=24  explicit_period=off  period=1  equ=P=C  opselect=C  inp2=PCIN>>17  opr=+  inp1=P  carry=CIN  dbl_ovrd=off  block_type=constant
  Constant6 : xbsIndex_r4/Constant  const=0  gui_display_data_type=Fixed-point  arith_type=Unsigned  n_bits=3  bin_pt=0  preci_type=Single  exp_width=8  frac_width=24  explicit_period=off  period=1  equ=P=C  opselect=C  inp2=PCIN>>17  opr=+  inp1=P  carry=CIN  dbl_ovrd=off  block_type=constant
  Constant7 : xbsIndex_r4/Constant  const=9  gui_display_data_type=Fixed-point  arith_type=Unsigned  n_bits=4  bin_pt=0  preci_type=Single  exp_width=8  frac_width=24  explicit_period=off  period=1  equ=P=C  opselect=C  inp2=PCIN>>17  opr=+  inp1=P  carry=CIN  dbl_ovrd=off  block_type=constant
  Convert1 : xbsIndex_r4/Convert  gui_display_data_type=Floating-point  arith_type=Floating-point  n_bits=16  bin_pt=14  float_type=Single  exp_bits=8  fraction_bits=24  quantization=Truncate  overflow=Wrap  en=off  latency=3  pipeline=off  dbl_ovrd=off  block_type=convert
  Convert4 : xbsIndex_r4/Convert  gui_display_data_type=Floating-point  arith_type=Floating-point  n_bits=16  bin_pt=14  float_type=Single  exp_bits=8  fraction_bits=24  quantization=Truncate  overflow=Wrap  en=off  latency=3  pipeline=off  dbl_ovrd=off  block_type=convert
  Convert5 : xbsIndex_r4/Convert  gui_display_data_type=Fixed-point  arith_type=Unsigned  n_bits=3  bin_pt=0  float_type=Single  exp_bits=8  fraction_bits=24  quantization=Truncate  overflow=Wrap  en=off  latency=0  pipeline=off  dbl_ovrd=off  block_type=convert
  Delay{1..3,11} (4 alike) : xbsIndex_r4/Delay  rst=off  infoeditControl=Selection of Reset will increase slice count due to use of real FFs and instead of SRLs  en=off  latency=1  reg_retiming=off  dbl_ovrd=off  block_type=delay
  Logical{,1..9} (10 alike) : xbsIndex_r4/Logical  logical_function=AND  inputs=2  en=off  latency=1  precision=Full  arith_type=Unsigned  n_bits=16  bin_pt=0  align_bp=on  dbl_ovrd=off  block_type=logical
  Mult1 : xbsIndex_r4/Mult  precision=Full  arith_type="Signed  (2's comp)"  n_bits=16  bin_pt=14  quantization=Truncate  overflow=Wrap  en=off  latency=3  use_behavioral_HDL=off  opt=Speed  use_embedded=on  optimum_pipeline=off  pipeline=on  dbl_ovrd=off  use_rpm=on  placement_style=Triangular  block_type=mult
  Mult3 : xbsIndex_r4/Mult  precision=Full  arith_type="Signed  (2's comp)"  n_bits=16  bin_pt=14  quantization=Truncate  overflow=Wrap  en=off  latency=3  use_behavioral_HDL=off  opt=Speed  use_embedded=on  optimum_pipeline=off  pipeline=on  dbl_ovrd=off  use_rpm=on  placement_style=Triangular  block_type=mult
  Mux{1,4..8,10..14} (11 alike) : xbsIndex_r4/Mux  inputs=2  en=off  latency=0  precision=Full  arith_type=Unsigned  n_bits=16  bin_pt=14  quantization=Truncate  overflow=Wrap  dbl_ovrd=off  block_type=mux
  Mux{2..3,9,15} (4 alike) : xbsIndex_r4/Mux  inputs=5  en=off  latency=1  precision=Full  arith_type=Unsigned  n_bits=16  bin_pt=14  quantization=Truncate  overflow=Wrap  dbl_ovrd=off  block_type=mux
  RSlice1 : xbsIndex_r4/Slice  nbits=4  boolean_output=off  mode=Upper Bit Location + Width  bit1=0  base1=MSB of Input  bit0=0  base0=LSB of Input  dbl_ovrd=off  block_type=slice
      settings: block_version=VER_STRING_GOES_HERE
  RSlice7 : xbsIndex_r4/Slice  nbits=7  boolean_output=off  mode=Lower Bit Location + Width  bit1=0  base1=MSB of Input  bit0=0  base0=LSB of Input  dbl_ovrd=off  block_type=slice
      settings: block_version=VER_STRING_GOES_HERE
  Reinterpret1 : xbsIndex_r4/Reinterpret  force_arith_type=on  arith_type="Signed  (2's comp)"  force_bin_pt=on  bin_pt=24  block_type=reinterpret
  Reinterpret2 : xbsIndex_r4/Reinterpret  force_arith_type=on  arith_type="Signed  (2's comp)"  force_bin_pt=on  bin_pt=24  block_type=reinterpret
  Relational{1..6,8..11,16..17} (12 alike) : xbsIndex_r4/Relational  mode=a=b  op_type=Bool  en=off  latency=0  dbl_ovrd=off  block_type=relational
  Scope1 : Scope  NumInputPorts=8
  Scope3 : Scope  NumInputPorts=10
  Shift1 : xbsIndex_r4/Shift  shift_dir=Right  shift_bits=5  en=off  latency=0  precision=Full  arith_type="Signed  (2's comp)"  n_bits=16  bin_pt=14  quantization=Truncate  overflow=Wrap  dbl_ovrd=off  block_type=shift
  Shift2 : xbsIndex_r4/Shift  shift_dir=Right  shift_bits=5  en=off  latency=0  precision=Full  arith_type="Signed  (2's comp)"  n_bits=16  bin_pt=14  quantization=Truncate  overflow=Wrap  dbl_ovrd=off  block_type=shift
  Single Port RAM1 : xbsIndex_r4/Single Port RAM  depth=96  initVector=ind_vol_4  distributed_mem=Block RAM  write_mode=Read After Write  rst=off  init_reg=0  en=off  optimize_latency=off  latency=1  optimize=Area  dbl_ovrd=off  simulation_type=fast_sim  block_type=spram
  Single Port RAM10 : xbsIndex_r4/Single Port RAM  depth=96  initVector=ind_vol_0  distributed_mem=Block RAM  write_mode=Read After Write  rst=off  init_reg=0  en=off  optimize_latency=off  latency=1  optimize=Area  dbl_ovrd=off  simulation_type=fast_sim  block_type=spram
  Single Port RAM2 : xbsIndex_r4/Single Port RAM  depth=96  initVector=ind_vol_3  distributed_mem=Block RAM  write_mode=Read After Write  rst=off  init_reg=0  en=off  optimize_latency=off  latency=1  optimize=Area  dbl_ovrd=off  simulation_type=fast_sim  block_type=spram
  Single Port RAM3 : xbsIndex_r4/Single Port RAM  depth=96  initVector=ind_vol_2  distributed_mem=Block RAM  write_mode=Read After Write  rst=off  init_reg=0  en=off  optimize_latency=off  latency=1  optimize=Area  dbl_ovrd=off  simulation_type=fast_sim  block_type=spram
  Single Port RAM4 : xbsIndex_r4/Single Port RAM  depth=96  initVector=ind_vol_1  distributed_mem=Block RAM  write_mode=Read After Write  rst=off  init_reg=0  en=off  optimize_latency=off  latency=1  optimize=Area  dbl_ovrd=off  simulation_type=fast_sim  block_type=spram
  Single Port RAM5 : xbsIndex_r4/Single Port RAM  depth=96  initVector=ind_vol_4  distributed_mem=Block RAM  write_mode=Read After Write  rst=off  init_reg=0  en=off  optimize_latency=off  latency=1  optimize=Area  dbl_ovrd=off  simulation_type=fast_sim  block_type=spram
  Single Port RAM6 : xbsIndex_r4/Single Port RAM  depth=96  initVector=ind_vol_3  distributed_mem=Block RAM  write_mode=Read After Write  rst=off  init_reg=0  en=off  optimize_latency=off  latency=1  optimize=Area  dbl_ovrd=off  simulation_type=fast_sim  block_type=spram
  Single Port RAM7 : xbsIndex_r4/Single Port RAM  depth=96  initVector=ind_vol_2  distributed_mem=Block RAM  write_mode=Read After Write  rst=off  init_reg=0  en=off  optimize_latency=off  latency=1  optimize=Area  dbl_ovrd=off  simulation_type=fast_sim  block_type=spram
  Single Port RAM8 : xbsIndex_r4/Single Port RAM  depth=96  initVector=ind_vol_1  distributed_mem=Block RAM  write_mode=Read After Write  rst=off  init_reg=0  en=off  optimize_latency=off  latency=1  optimize=Area  dbl_ovrd=off  simulation_type=fast_sim  block_type=spram
  Single Port RAM9 : xbsIndex_r4/Single Port RAM  depth=96  initVector=ind_vol_0  distributed_mem=Block RAM  write_mode=Read After Write  rst=off  init_reg=0  en=off  optimize_latency=off  latency=1  optimize=Area  dbl_ovrd=off  simulation_type=fast_sim  block_type=spram
  Slice1 : xbsIndex_r4/Slice  nbits=5  boolean_output=off  mode=Lower Bit Location + Width  bit1=0  base1=LSB of Input  bit0=0  base0=LSB of Input  dbl_ovrd=off  block_type=slice
  Slice3 : xbsIndex_r4/Slice  nbits=2  boolean_output=off  mode=Upper Bit Location + Width  bit1=0  base1=MSB of Input  bit0=0  base0=LSB of Input  dbl_ovrd=off  block_type=slice
  const : xbsIndex_r4/Constant  const=0  gui_display_data_type=Fixed-point  arith_type=Unsigned  n_bits=7  bin_pt=0  preci_type=Single  exp_width=8  frac_width=24  explicit_period=on  period=1  equ=P=C  opselect=C  inp2=PCIN>>17  opr=+  inp1=P  carry=CIN  dbl_ovrd=off  block_type=constant
      settings: block_version=VER_STRING_GOES_HERE
  ind_vol : xbsIndex_r4/Constant  const=CMD_ind_vol  gui_display_data_type=Fixed-point  arith_type=Unsigned  n_bits=8  bin_pt=0  preci_type=Single  exp_width=8  frac_width=24  explicit_period=on  period=1  equ=P=C  opselect=C  inp2=PCIN>>17  opr=+  inp1=P  carry=CIN  dbl_ovrd=off  block_type=constant
      settings: block_version=VER_STRING_GOES_HERE
  x : xbsIndex_r4/Constant  const=8000000  gui_display_data_type=Fixed-point  arith_type=Unsigned  n_bits=24  bin_pt=0  preci_type=Single  exp_width=8  frac_width=24  explicit_period=on  period=1  equ=P=C  opselect=C  inp2=PCIN>>17  opr=+  inp1=P  carry=CIN  dbl_ovrd=off  block_type=constant
      settings: block_version=VER_STRING_GOES_HERE
  x1 : xbsIndex_r4/Constant  const=8000000  gui_display_data_type=Fixed-point  arith_type=Unsigned  n_bits=24  bin_pt=0  preci_type=Single  exp_width=8  frac_width=24  explicit_period=on  period=1  equ=P=C  opselect=C  inp2=PCIN>>17  opr=+  inp1=P  carry=CIN  dbl_ovrd=off  block_type=constant
      settings: block_version=VER_STRING_GOES_HERE
  z1 : xbsIndex_r4/Delay  rst=off  infoeditControl=Selection of Reset will increase slice count due to use of real FFs and instead of SRLs  en=off  latency=11  reg_retiming=on  dbl_ovrd=off  block_type=delay
      settings: block_version=8.2-EVAL
  z{2,4..13,15,17,20..23,25,27,30..34} (24 alike) : xbsIndex_r4/Delay  rst=off  infoeditControl=Selection of Reset will increase slice count due to use of real FFs and instead of SRLs  en=off  latency=1  reg_retiming=on  dbl_ovrd=off  block_type=delay
      settings: block_version=8.2-EVAL
  z14 : xbsIndex_r4/Delay  rst=off  infoeditControl=Selection of Reset will increase slice count due to use of real FFs and instead of SRLs  en=off  latency=2  reg_retiming=on  dbl_ovrd=off  block_type=delay
      settings: block_version=8.2-EVAL
  z16 : xbsIndex_r4/Delay  rst=off  infoeditControl=Selection of Reset will increase slice count due to use of real FFs and instead of SRLs  en=off  latency=7  reg_retiming=on  dbl_ovrd=off  block_type=delay
      settings: block_version=8.2-EVAL
  z18 : xbsIndex_r4/Delay  rst=off  infoeditControl=Selection of Reset will increase slice count due to use of real FFs and instead of SRLs  en=off  latency=7  reg_retiming=on  dbl_ovrd=off  block_type=delay
      settings: block_version=8.2-EVAL
  z19 : xbsIndex_r4/Delay  rst=off  infoeditControl=Selection of Reset will increase slice count due to use of real FFs and instead of SRLs  en=off  latency=11  reg_retiming=on  dbl_ovrd=off  block_type=delay
      settings: block_version=8.2-EVAL
  z24 : xbsIndex_r4/Delay  rst=off  infoeditControl=Selection of Reset will increase slice count due to use of real FFs and instead of SRLs  en=off  latency=2  reg_retiming=on  dbl_ovrd=off  block_type=delay
      settings: block_version=8.2-EVAL
  z28 : xbsIndex_r4/Delay  rst=off  infoeditControl=Selection of Reset will increase slice count due to use of real FFs and instead of SRLs  en=off  latency=4  reg_retiming=on  dbl_ovrd=off  block_type=delay
      settings: block_version=8.2-EVAL
  z3 : xbsIndex_r4/Delay  rst=off  infoeditControl=Selection of Reset will increase slice count due to use of real FFs and instead of SRLs  en=off  latency=4  reg_retiming=on  dbl_ovrd=off  block_type=delay
      settings: block_version=8.2-EVAL
  vol : Outport  VectorParamsAs1DForOutWhenUnconnected=off
  Vol_stuk : Outport  Port=2  VectorParamsAs1DForOutWhenUnconnected=off
  wires:
  z17/1 -> z18/1
  Delay1/1 -> Reinterpret1/1
  Delay11/1 -> vol/1
  Convert4/1 -> Delay11/1
  Reinterpret1/1 -> Convert4/1
  z15/1 -> Mux3/2
  z13/1 -> Mux2/2, Mux3/3
  z12/1 -> Mux3/4, Mux2/3
  z11/1 -> Mux2/4, Mux3/5
  z10/1 -> Mux2/5
  AddSub6/1 -> Delay1/1
  z3/1 -> AddSub6/2
  z14/1 -> z3/1
  z2/1 -> AddSub6/1
  Mult3/1 -> z2/1
  z1/1 -> Mult3/2
  Shift2/1 -> Mult3/1
  AddSub5/1 -> Shift2/1
  Mux3/1 -> AddSub5/2, z14/1
  Mux2/1 -> AddSub5/1
  Constant1/1 -> Mux3/6
  Constant10/1 -> Mux2/6
  Slice3/1 -> Convert5/1
  Convert5/1 -> Mux1/2
  Relational16/1 -> Mux1/1
  Constant2/1 -> Mux1/3
  const/1 -> Relational16/2
  Single Port RAM5/1 -> z10/1
  Single Port RAM6/1 -> z11/1
  Single Port RAM7/1 -> z12/1
  Single Port RAM9/1 -> z15/1
  Single Port RAM8/1 -> z13/1
  Mux1/1 -> z17/1
  force_vol/1 -> Slice3/1, Slice1/1, Relational16/1
  m_en/1 -> Relational17/1
  m_addr/1 -> RSlice7/1, RSlice1/1
  Mux14/1 -> Single Port RAM9/1
  Logical4/1 -> Mux14/1, Single Port RAM9/3
  addr_ind_vol/1 -> z4/1
  Mux12/1 -> Single Port RAM7/1
  Mux13/1 -> Single Port RAM8/1
  Mux11/1 -> Single Port RAM6/1
  Logical2/1 -> Mux12/1, Single Port RAM7/3
  ind_vol/1 -> Relational17/2
  Logical1/1 -> Mux11/1, Single Port RAM6/3
  Logical/1 -> Single Port RAM5/3, Mux10/1
  Logical3/1 -> Single Port RAM8/3, Mux13/1
  Mux10/1 -> Single Port RAM5/1
  z4/1 -> z16/1
  z5/1 -> Mux10/2
  z6/1 -> Mux11/2
  z7/1 -> Mux12/2
  z8/1 -> Mux13/2
  z9/1 -> Mux14/2
  Constant/1 -> Relational1/2
  Constant3/1 -> Relational2/2
  Constant4/1 -> Relational3/2
  Constant5/1 -> Relational4/2
  Constant6/1 -> Relational5/2
  Relational1/1 -> Logical/2
  Relational2/1 -> Logical1/2
  Relational3/1 -> Logical2/2
  Relational4/1 -> Logical3/2
  Relational5/1 -> Logical4/2
  Mux7/1 -> Single Port RAM4/1
  Mux9/1 -> AddSub1/1
  Constant14/1 -> Relational11/2
  Relational11/1 -> Logical9/2
  Mux15/1 -> AddSub1/2, z24/1
  Single Port RAM10/1 -> z25/1
  z22/1 -> Mux15/4, Mux9/3
  Logical9/1 -> Mux8/1, Single Port RAM10/3
  Relational8/1 -> Logical6/2
  z34/1 -> Mux8/2
  Mult1/1 -> z27/1
  Relational9/1 -> Logical7/2
  Constant7/1 -> Relational6/2
  Logical7/1 -> Mux6/1, Single Port RAM3/3
  RSlice1/1 -> Relational2/1, Relational3/1, Relational4/1, Relational8/1, Relational9/1, Relational10/1, Relational11/1, Relational6/1, Relational5/1, Relational1/1
  Relational17/1 -> Logical1/1, Logical2/1, Logical3/1, Logical6/1, Logical7/1, Logical8/1, Logical9/1, Logical5/1, Logical4/1, Logical/1
  Mux8/1 -> Single Port RAM10/1
  Relational6/1 -> Logical5/2
  Constant12/1 -> Relational9/2
  Constant11/1 -> Relational8/2
  z32/1 -> Mux6/2
  z27/1 -> AddSub2/1
  Constant8/1 -> Mux15/6
  RSlice7/1 -> Mux10/3, Mux13/3, Mux7/3, Mux8/3, Mux6/3, Mux5/3, Mux4/3, Mux14/3, Mux12/3, Mux11/3
  z20/1 -> Mux9/5
  Constant9/1 -> Mux9/6
  Mux4/1 -> Single Port RAM1/1
  dat_in/1 -> Single Port RAM5/2, Single Port RAM8/2, Single Port RAM1/2, Single Port RAM4/2, Single Port RAM10/2, Single Port RAM3/2, Single Port RAM2/2, Single Port RAM9/2, Single Port RAM7/2, Single Port RAM6/2
  Logical5/1 -> Single Port RAM1/3, Mux4/1
  z30/1 -> Mux4/2
  z19/1 -> Mult1/2
  z24/1 -> z28/1
  Slice1/1 -> z19/1, z1/1
  Logical6/1 -> Mux5/1, Single Port RAM2/3
  Single Port RAM1/1 -> z20/1
  Mux5/1 -> Single Port RAM2/1
  Single Port RAM3/1 -> z22/1
  z33/1 -> Mux7/2
  Shift1/1 -> Mult1/1
  Delay3/1 -> Vol_stuk/1
  z25/1 -> Mux15/2
  Constant13/1 -> Relational10/2
  Single Port RAM4/1 -> z23/1
  Reinterpret2/1 -> Convert1/1
  Relational10/1 -> Logical8/2
  z28/1 -> AddSub2/2
  z23/1 -> Mux9/2, Mux15/3
  AddSub1/1 -> Shift1/1
  z31/1 -> Mux5/2
  Convert1/1 -> Delay3/1
  z16/1 -> z5/1, z6/1, z8/1, z30/1, z31/1, z33/1, z34/1, z32/1, z9/1, z7/1
  Mux6/1 -> Single Port RAM3/1
  z21/1 -> Mux9/4, Mux15/5
  z18/1 -> Mux2/1, Mux9/1, Mux15/1, Mux3/1
  Single Port RAM2/1 -> z21/1
  Logical8/1 -> Single Port RAM4/3, Mux7/1
  Delay2/1 -> Reinterpret2/1
  AddSub2/1 -> Delay2/1
